simulink library "SEN_GYR"  (Simulink 10.2)
settings: Solver=VariableStepAuto  StartTime=0.0  StopTime=10.0  RelTol=1e-3
undefined symbols (not defined in the file): SEN_GYR_par
libraries: simulink x1
settings Model: Creator=dbell44  LastModifiedBy=dbell44

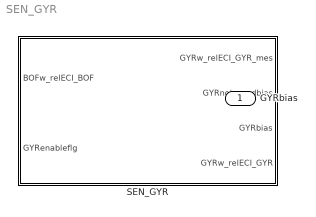
== system SEN_GYR ==
  SEN_GYR : Subsystem
  GYRbias : Outport  PortDimensions=3  VectorParamsAs1DForOutWhenUnconnected=off

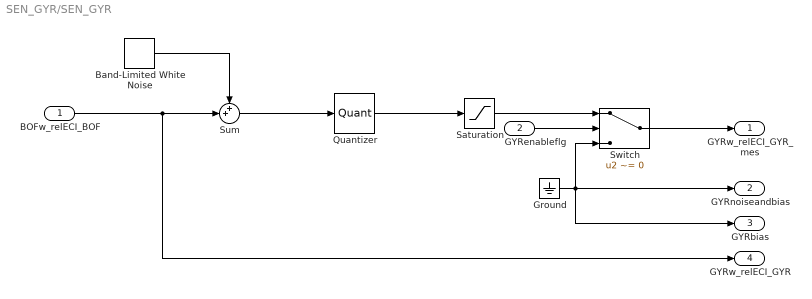
== system SEN_GYR/SEN_GYR ==
  BOFw_relECI_BOF : Inport
  GYRenableflg : Inport  Port=2
  Band-Limited White Noise : simulink/Sources/Band-Limited White Noise  Cov=SEN_GYR_par.noise_power  Ts=1/SEN_GYR_par.sample_rate  seed=randi([1 243453])
  Ground : Ground
  Quantizer : Quantizer  QuantizationInterval=SEN_GYR_par.sensitivity  LinearizeAsGain=off
  Saturation : Saturate  UpperLimit=SEN_GYR_par.full_scale_range  LowerLimit=-SEN_GYR_par.full_scale_range
  Sum : Sum  Inputs=++|
  Switch : Switch  Criteria=u2 ~= 0
  GYRw_relECI_GYR_mes : Outport  PortDimensions=3  VectorParamsAs1DForOutWhenUnconnected=off
  GYRnoiseandbias : Outport  Port=2  PortDimensions=3  VectorParamsAs1DForOutWhenUnconnected=off
  GYRbias : Outport  Port=3  PortDimensions=3  VectorParamsAs1DForOutWhenUnconnected=off
  GYRw_relECI_GYR : Outport  Port=4  PortDimensions=3  VectorParamsAs1DForOutWhenUnconnected=off
  wires:
  Band-Limited White Noise/1 -> Sum/1
  Sum/1 -> Quantizer/1
  Quantizer/1 -> Saturation/1
  BOFw_relECI_BOF/1 -> GYRw_relECI_GYR/1, Sum/2
  Saturation/1 -> Switch/1
  GYRenableflg/1 -> Switch/2
  Ground/1 -> GYRnoiseandbias/1, Switch/3, GYRbias/1
  Switch/1 -> GYRw_relECI_GYR_mes/1
